simulink model "IntegrationTestSim"  (R2018b)
settings: Solver=ode45  StartTime=0.0  StopTime=600  RelTol=1e-3  EnableMultiTasking=on
values from neighbouring files (symbols this model uses):
  enableHorzMan = 1    [IntegrationTestClass.m]
  enableVertMan = 0    [IntegrationTestClass.m]
  ignorePrevAlert = 1    [IntegrationTestClass.m]
  sim_sampleTime = 0.1    [IntegrationTestClass.m]
  uasSensorSelected = 1    [IntegrationTestClass.m]
  uasSurveillance_sampleTime = 0.1    [IntegrationTestClass.m]
undefined symbols (not defined in the file or in its folder): ac1dyn_alt0_ft, ac1dyn_lat0_rad, ac1dyn_lon0_rad, daa_turnRate_dps, daa_vertRate_fpm, dh_flag, dh_ftps, dpsi_flag, dpsi_radps, uasPilot_altitudeK, uasPilot_altitudeOffset, uasPilot_altitudeTheta, uasPilot_coordDelayK, uasPilot_coordDelayMin, uasPilot_coordDelayTheta, uasPilot_desiredTurnRate_dps, uasPilot_desiredVertRate_ftpm, uasPilot_deterministicMode, uasPilot_dt_s, uasPilot_executionDelayMin, uasPilot_executionDelayMu, uasPilot_initialDelayMin, uasPilot_initialDelayMu, uasPilot_maxRelativeHdg, uasPilot_meanUpdateTimes, uasPilot_mentalFilter_climbThresh_fps, uasPilot_mentalFilter_numSamp, uasPilot_mentalFilter_turnThresh_rad, uasPilot_minUpdateTimes, uasPilot_operatorEnabled, uasPilot_probDescend, uasPilot_probFollowMinDev, uasPilot_probLeftTurn, uasPilot_probTurn, uasPilot_reducedClimbAlt_ft, uasPilot_reducedTurnAngle_deg, uasPilot_seedChoose, uasPilot_seedCoordDelay, uasPilot_seedExecutionDelay, uasPilot_seedInitialDelay, uasPilot_seedTurn, uasPilot_seedUpdate, uasPilot_seedVertical, uasPilot_triggerLevel, uasPilot_turnK, uasPilot_turnOffset, uasPilot_turnTheta
libraries: simulink x4, BasicAircraftDynamicsBlock x3, NominalTrajectory x2, FlattenAircraftEstimateBus x2, PerfectSurveillanceBlock x2, sph2cart x2, DaidalusV201Block x1, HysteresisFilterBlock x1, MofNFilterBlock x1, CommonMetricsBlock x1, SLoWCBlock x1, WellClearMetricsBlock x1
(part 2 of 3)

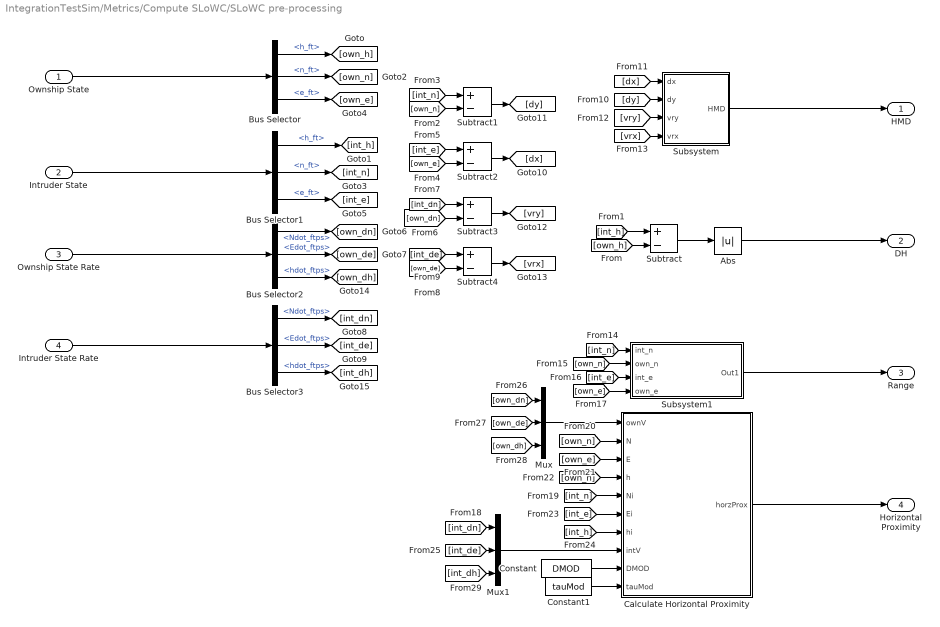
== system IntegrationTestSim/Metrics/Compute SLoWC/SLoWC pre-processing ==
  Ownship State : Inport
  Intruder State : Inport  Port=2
  Ownship State Rate : Inport  Port=3
  Intruder State Rate : Inport  Port=4
  Abs : Abs
  Bus Selector : BusSelector  OutputSignals=h_ft,n_ft,e_ft
  Bus Selector1 : BusSelector  OutputSignals=h_ft,n_ft,e_ft
  Bus Selector2 : BusSelector  OutputSignals=Ndot_ftps,Edot_ftps,hdot_ftps
  Bus Selector3 : BusSelector  OutputSignals=Ndot_ftps,Edot_ftps,hdot_ftps
  Calculate Horizontal Proximity : MATLAB Function  TreatAsAtomicUnit=on
  Constant : Constant  Value=DMOD
  Constant1 : Constant  Value=tauMod
  Mux : Mux  Inputs=3
  Mux1 : Mux  Inputs=3
  Subsystem : Subsystem
  Subsystem1 : Subsystem
  Subtract{,1..4} (5 alike) : Sum  Inputs=+-
  HMD : Outport
  DH : Outport  Port=2
  Range : Outport  Port=3
  Horizontal Proximity : Outport  Port=4
  wires:
  Subtract/1 -> Abs/1
  [own_dh] -> Mux/3
  Bus Selector/1 -> [own_h]  "<h_ft>"
  [own_dn] -> Subtract3/2
  Bus Selector1/3 -> [int_e]  "<e_ft>"
  [int_n] -> Calculate Horizontal Proximity/5(Ni)
  Bus Selector3/3 -> [int_dh]  "<hdot_ftps>"
  [int_h] -> Calculate Horizontal Proximity/7(hi)
  [int_e] -> Subtract2/1
  [own_h] -> Subtract/2
  Intruder State/1 -> Bus Selector1/1
  [own_n] -> Subtract1/2
  Constant/1 -> Calculate Horizontal Proximity/9(DMOD)
  [own_e] -> Subtract2/2
  [int_dh] -> Mux1/3
  Subtract4/1 -> [vrx]
  [int_h] -> Subtract/1
  Bus Selector1/1 -> [int_h]  "<h_ft>"
  [vry] -> Subsystem/3(vry)
  [own_n] -> Calculate Horizontal Proximity/2(N)
  Bus Selector3/1 -> [int_dn]  "<Ndot_ftps>"
  Subtract2/1 -> [dx]
  Bus Selector1/2 -> [int_n]  "<n_ft>"
  Bus Selector/2 -> [own_n]  "<n_ft>"
  Subtract3/1 -> [vry]
  [int_e] -> Subsystem1/3(int_e)
  [own_de] -> Mux/2
  Mux1/1 -> Calculate Horizontal Proximity/8(intV)
  Subtract1/1 -> [dy]
  [own_h] -> Calculate Horizontal Proximity/4(h)
  [dy] -> Subsystem/2(dy)
  [own_n] -> Subsystem1/2(own_n)
  [int_dn] -> Mux1/1
  Subsystem/1(HMD) -> HMD/1
  Bus Selector2/2 -> [own_de]  "<Edot_ftps>"
  [int_n] -> Subtract1/1
  Bus Selector2/3 -> [own_dh]  "<hdot_ftps>"
  [int_de] -> Subtract4/1
  Constant1/1 -> Calculate Horizontal Proximity/10(tauMod)
  Bus Selector/3 -> [own_e]  "<e_ft>"
  Subsystem1/1(Out1) -> Range/1
  [int_n] -> Subsystem1/1("int_n ")
  [int_e] -> Calculate Horizontal Proximity/6(Ei)
  [own_de] -> Subtract4/2
  Bus Selector3/2 -> [int_de]  "<Edot_ftps>"
  Mux/1 -> Calculate Horizontal Proximity/1(ownV)
  [dx] -> Subsystem/1("dx ")
  [int_dn] -> Subtract3/1
  Intruder State Rate/1 -> Bus Selector3/1
  [vrx] -> Subsystem/4(vrx)
  [own_dn] -> Mux/1
  Bus Selector2/1 -> [own_dn]  "<Ndot_ftps>"
  Abs/1 -> DH/1
  [own_e] -> Calculate Horizontal Proximity/3(E)
  Calculate Horizontal Proximity/1(horzProx) -> Horizontal Proximity/1
  Ownship State/1 -> Bus Selector/1
  [int_de] -> Mux1/2
  [own_e] -> Subsystem1/4(own_e)
  Ownship State Rate/1 -> Bus Selector2/1

== system IntegrationTestSim/Pilot/Format Maneuver As AircraftCommand/Get Previous Command ==
  Cmd In : Inport
  Nominal Cmd : Inport  Port=2
  Maneuver Flag : Inport  Port=3
  Data Type Conversion : DataTypeConversion  OutDataTypeStr=double
  Memory : Memory  InheritSampleTime=on
  Switch : Switch  Criteria=u2 > Threshold
  Cmd Out : Outport
  wires:
  Maneuver Flag/1 -> Memory/1
  Memory/1 -> Data Type Conversion/1
  Nominal Cmd/1 -> Switch/3
  Switch/1 -> Cmd Out/1
  Cmd In/1 -> Switch/1
  Data Type Conversion/1 -> Switch/2

== system IntegrationTestSim/Pilot/Format Maneuver As AircraftCommand/Horizontal Maneuver ==
  Command In : Inport
  Maneuver : Inport  Port=2
  Own State : Inport  Port=3
  Maneuver Flag : Inport  Port=4  OutDataTypeStr=boolean
  Bus Selector : BusSelector  OutputSignals=type
  Compare To Constant : simulink/Logic and Bit Operations/Compare To Constant  relop===  const=1  OutDataTypeStr=boolean
  Data Type Conversion1 : DataTypeConversion  OutDataTypeStr=double
  Logical Operator : Logic  AllPortsSameDT=off  OutDataTypeStr=boolean
  Set Desired Turn Rate : Subsystem
  Switch : Switch  Criteria=u2 > Threshold
  Cmd Out : Outport
  wires:
  Bus Selector/1 -> Compare To Constant/1  "<type>"
  Maneuver/1 -> Set Desired Turn Rate/2(Maneuver Magnitude), Bus Selector/1
  Own State/1 -> Set Desired Turn Rate/3(Own State)
  Maneuver Flag/1 -> Data Type Conversion1/1
  Logical Operator/1 -> Switch/2
  Command In/1 -> Switch/3, Set Desired Turn Rate/1(Cmd In)
  Data Type Conversion1/1 -> Logical Operator/1
  Compare To Constant/1 -> Logical Operator/2
  Set Desired Turn Rate/1(Cmd Out) -> Switch/1
  Switch/1 -> Cmd Out/1

== system IntegrationTestSim/Pilot/Format Maneuver As AircraftCommand/Vertical Maneuver ==
  Command In : Inport
  Maneuver : Inport  Port=2
  Own State : Inport  Port=3
  Maneuver Flag : Inport  Port=4  OutDataTypeStr=boolean
  UAS Nominal Traj : Inport  Port=5
  Bus Selector1 : BusSelector  OutputSignals=dh_ftps,h_ft
  Bus Selector : BusSelector  OutputSignals=type
  Compare To Constant : simulink/Logic and Bit Operations/Compare To Constant  relop===  const=2  OutDataTypeStr=boolean
  Data Type Conversion1 : DataTypeConversion  OutDataTypeStr=double
  Logical Operator : Logic  AllPortsSameDT=off  OutDataTypeStr=boolean
  Scope : Scope
  Scope1 : Scope
  Set Desired Vertical Rate : Subsystem
  Switch : Switch  Criteria=u2 > Threshold
  Cmd Out : Outport
  wires:
  Bus Selector/1 -> Compare To Constant/1  "<type>"
  Maneuver Flag/1 -> Data Type Conversion1/1
  Switch/1 -> Cmd Out/1
  Data Type Conversion1/1 -> Logical Operator/1
  Compare To Constant/1 -> Logical Operator/2
  Command In/1 -> Set Desired Vertical Rate/1(Cmd In), Switch/3
  Set Desired Vertical Rate/1(Cmd Out) -> Switch/1
  UAS Nominal Traj/1 -> Bus Selector1/1
  Bus Selector1/2 -> Scope/1  "<h_ft>"
  Own State/1 -> Set Desired Vertical Rate/2(Own State)
  Maneuver/1 -> Set Desired Vertical Rate/3(Maneuver), Bus Selector/1
  Bus Selector1/1 -> Set Desired Vertical Rate/4(dh_ftps)  "<dh_ftps>"
  Logical Operator/1 -> Scope1/1, Switch/2

== system IntegrationTestSim/Pilot/Trigger/Filter Alerts ==
  Alert Level In : Inport
  Constant6 : Constant  Value=trigger_level
  Relational Operator : RelationalOperator  OutDataTypeStr=boolean  RndMeth=Nearest
  Trigger : Outport
  wires:
  Relational Operator/1 -> Trigger/1
  Constant6/1 -> Relational Operator/2
  Alert Level In/1 -> Relational Operator/1

== system IntegrationTestSim/Surveillance Source/Subsystem/EOIR Parameteric Model ==
  Intruder Aircraft State : Inport
  Intruder Aircraft State Rate : Inport  Port=2
  Ownship Aircraft State : Inport  Port=3
  Ownship Aircraft State Rate : Inport  Port=4
  EOIR Parametric Model : EOIRParametricModelBlock/EOIR Parametric Model  dt_s=ac1IntEOIR_dt_s  lat0_rad=ac1dyn_lat0_rad  lon0_rad=ac1dyn_lon0_rad  alt0_ft=ac1dyn_alt0_ft  sns_max_range_ft=ac1IntEOIR_sns_max_range_ft  sns_for_azimuth_deg=ac1IntEOIR_sns_for_azimuth_deg  sns_for_elevation_deg=ac1IntEOIR_sns_for_elevation_deg  rng_random_stddev_ft=ac1IntEOIR_rng_random_stddev_ft  rng_bias_ft=ac1IntEOIR_rng_bias_ft  rng_tau_s=ac1IntEOIR_rng_tau_s  seed1=ac1IntEOIR_seed1  rng_std_dev_gain=ac1IntEOIR_rng_std_dev_gain  rng_bias_switch=ac1IntEOIR_rng_bias_switch  coloredNoiseFlag=0  az_random_stddev_rad=ac1IntEOIR_az_random_stddev_rad  az_bias_rad=ac1IntEOIR_az_bias_rad  az_tau_s=ac1IntEOIR_az_tau_s  seed2=ac1IntEOIR_seed2  el_random_stddev_rad=ac1IntEOIR_el_random_stddev_rad  el_bias_rad=ac1IntEOIR_el_bias_rad  el_tau_s=ac1IntEOIR_el_tau_s  seed3=ac1IntEOIR_seed3  rngdot_random_stddev_ftps=ac1IntEOIR_rngdot_random_stddev_ftps  rngdot_bias_ftps=ac1IntEOIR_rngdot_bias_ftps  rngdot_tau_s=ac1IntEOIR_rngdot_tau_s  seed4=ac1IntEOIR_seed4  rngdot_std_dev_gain=ac1IntEOIR_rngdot_std_dev_gain  rngdot_delay_s=ac1IntEOIR_rngdot_delay_s  azdot_random_stddev_radps=ac1IntEOIR_azdot_random_stddev_radps  azdot_bias_radps=ac1IntEOIR_azdot_bias_radps  azdot_tau_s=ac1IntEOIR_azdot_tau_s  seed5=ac1IntEOIR_seed5  eldot_random_stddev_radps=ac1IntEOIR_eldot_random_stddev_radps  eldot_bias_radps=ac1IntEOIR_eldot_bias_radps  eldot_tau_s=ac1IntEOIR_eldot_tau_s  seed6=ac1IntEOIR_seed6  covRAE=ac1IntEOIR_reported_errorCovRAE
  Terminator : Terminator
  Intruder AircraftEstimate : Outport
  wires:
  Ownship Aircraft State Rate/1 -> EOIR Parametric Model/4
  Intruder Aircraft State/1 -> EOIR Parametric Model/1
  EOIR Parametric Model/1 -> Intruder AircraftEstimate/1
  Intruder Aircraft State Rate/1 -> EOIR Parametric Model/2
  Ownship Aircraft State/1 -> EOIR Parametric Model/3
  EOIR Parametric Model/2 -> Terminator/1

== system IntegrationTestSim/Surveillance Source/Subsystem/Perfect Surveillance ==
  Intruder Aircraft State : Inport
  Intruder Aircraft State Rate : Inport  Port=2
  Intruder Sensor - Perfect Surveillance : PerfectSurveillanceBlock/Perfect Surveillance  Description=|  dt=ac1IntPerfSurv_surveillanceSampletime_s
      | Documentation for Perfect Observation Block                                                                                                                                                                                                                                                                                                                                                                                                          
      |                                                                                                                                                                                                                                                                                                                                                                                                                                                      
      | Description:  The perfect observation block, also known as a perfect                                                                                                                                                                                                                                                                                                                                                                                 
      | surveillance block, receives an Aircraft State, nominally from a Basic                                                                                                                                                                                                                                                                                                                                                                               
      | Aircraft Dynamics block, and outputs an Aircraft Estimate.  The Aircraft                                                                                                                                                                                                                                                                                                                                                                             
      | State that is received as input consists of Latitude, Longitude, and                                                                                                                                                                                                                                                                                                                                                                                 
      | Altitude state information as well as the aircraft position in local                                                                                                                                                                                                                                                                                                                                                                                 
      | coordinates in units of feet for north, east, and height.  The Aircraft                                                                                                                                                                                                                                                                                                                                                                              
      | Estimate outputs consist of estimates for the aircraft Latitude, Longitude, and Altitude, the east, north up position, and sensor covariance.  For perfect surveillance, the covariance estimates are all set to zero as default.  In addition, "time of validity" and a Boolean flag for the sensor report, "is Valid", are outputted as part of the Aircraft Estimate.                                                                             
      |                                                                                                                                                                                                                                                                                                                                                                                                                                                      
      | The initial perfect surveillance block developed receives the aircraft state information from the "AC2 - Basic Aircraft Dynamics" block within the "nominalEncounter" study.  Since the expected output from the AC1 and AC2 aircraft states have slightly different output parameters than what is provided from the perfect surveillance block (i.e., covariance estimates, isValid, and time of validity), the perfect surveillance block         
      | AircraftEstimate output has been left disconnected.                                                                                                                                                                                                                                                                                                                                                                                                  
      |                                                                                                                                                                                                                                                                                                                                                                                                                                                      
      | The initial unit test performed for this perfect observation block was to                                                                                                                                                                                                                                                                                                                                                                            
      | run the nominalEncounter study and to ensure that the simulation completes and no exceptions are encountered.  This unit test was successful (other than receiving a warning that the output of the perfect surveillance block is not connected, which was expected).  A more comprehensive future unit test would be to evaluate the position inputs and compare them with the position outputs to ensure that they are consistent with one another.
  Terminator : Terminator
  Intruder AircraftEstimate : Outport
  wires:
  Intruder Aircraft State/1 -> Intruder Sensor - Perfect Surveillance/1
  Intruder Sensor - Perfect Surveillance/2 -> Terminator/1
  Intruder Aircraft State Rate/1 -> Intruder Sensor - Perfect Surveillance/2
  Intruder Sensor - Perfect Surveillance/1 -> Intruder AircraftEstimate/1

== system IntegrationTestSim/Surveillance Source/Subsystem/SC-228 ADSB Model ==
  Intruder Aircraft State : Inport
  Intruder Aircraft State Rate : Inport  Port=2
  Owship Aircraft State : Inport  Port=3
  SC-228 Sensor Model: ADS-B : ADSB_Block/SC-228 Sensor Model: ADS-B  var_prefix=int_  dt_s=uas_adsb_dt_s  lat0_rad=ac1dyn_lat0_rad  lon0_rad=ac1dyn_lon0_rad  alt0_ft=ac1dyn_alt0_ft  avionicsSeed=uas_adsb_avionicsSeed  N_random_stddev_ft=uas_adsb_N_random_stddev_ft  N_bias_ft=uas_adsb_N_bias_ft  N_tau_s=uas_adsb_N_tau_s  seed1=uas_adsb_seed1  E_random_stddev_ft=uas_adsb_E_random_stddev_ft  E_bias_ft=uas_adsb_E_bias_ft  E_tau_s=uas_adsb_E_tau_s  seed2=uas_adsb_seed2  Ndot_random_stddev_ftps=uas_adsb_Ndot_random_stddev_ftps  Ndot_bias_ftps=uas_adsb_Ndot_bias_ftps  Ndot_tau_s=uas_adsb_Ndot_tau_s  seed5=uas_adsb_seed5  Edot_random_stddev_ftps=uas_adsb_Edot_random_stddev_ftps  Edot_bias_ftps=uas_adsb_Edot_bias_ftps  Edot_tau_s=uas_adsb_Edot_tau_s  seed6=uas_adsb_seed6  covNED=uas_adsb_reported_errorCovNED  perfect=uas_adsb_usePerfectAlt  seed3=uas_adsb_seed3  seed4=uas_adsb_seed4  altQuant_ft=uas_adsb_altQuant_ft  seed7=uas_adsb_seed7  sns_max_range_ft=uas_adsb_sns_max_range_ft  probOneHit_3sec=uas_adsb_probOneHit_3sec  probOneHit_7sec=uas_adsb_probOneHit_7sec  randProbSeed=uas_adsb_randProbSeed  rangeThreshold_ft=uas_adsb_rangeThreshold_ft
  Terminator : Terminator
  Intruder AircraftEstimate : Outport
  wires:
  Owship Aircraft State/1 -> SC-228 Sensor Model: ADS-B/3
  SC-228 Sensor Model: ADS-B/2 -> Terminator/1
  Intruder Aircraft State Rate/1 -> SC-228 Sensor Model: ADS-B/2
  Intruder Aircraft State/1 -> SC-228 Sensor Model: ADS-B/1
  SC-228 Sensor Model: ADS-B/1 -> Intruder AircraftEstimate/1

== system IntegrationTestSim/Surveillance Source/Subsystem/SC-228 ADSB Model (Tracked) ==
  Intruder Aircraft State : Inport
  Intruder Aircraft State Rate : Inport  Port=2
  Ownship Aircraft State : Inport  Port=3
  SC-228 Sensor Model: ADS-B (Tracked) : Tracked_ADSB_Block/SC-228 Sensor Model: ADS-B (Tracked)  var_prefix=int_  dt_s=uas_adsb_trckd_dt_s  lat0_rad=ac1dyn_lat0_rad  lon0_rad=ac1dyn_lon0_rad  alt0_ft=ac1dyn_alt0_ft  avionicsSeed=uas_adsb_trckd_avionicsSeed  N_random_stddev_ft=uas_adsb_trckd_N_stddev_ft  N_bias_ft=uas_adsb_trckd_N_bias_ft  N_tau_s=uas_adsb_trckd_N_tau_s  seed1=uas_adsb_trckd_seed1  E_random_stddev_ft=uas_adsb_trckd_E_stddev_ft  E_bias_ft=uas_adsb_trckd_E_bias_ft  E_tau_s=uas_adsb_trckd_E_tau_s  seed2=uas_adsb_trckd_seed2  Ndot_random_stddev_ftps=uas_adsb_trckd_Ndot_stddev_ftps  Ndot_bias_ftps=uas_adsb_trckd_Ndot_bias_ftps  Ndot_tau_s=uas_adsb_trckd_Ndot_tau_s  seed5=uas_adsb_trckd_seed5  Edot_random_stddev_ftps=uas_adsb_trckd_Edot_stddev_ftps  Edot_bias_ftps=uas_adsb_trckd_Edot_bias_ftps  Edot_tau_s=uas_adsb_trckd_Edot_tau_s  seed6=uas_adsb_trckd_seed6  covNED=uas_adsb_trckd_reported_errorCovNED  seed3=uas_adsb_trckd_seed3  seed4=uas_adsb_trckd_seed4  altQuant_ft=uas_adsb_trckd_altQuant_ft  seed7=uas_adsb_trckd_seed7  sns_max_range_ft=uas_adsb_trckd_sns_max_range_ft  probOneHit_3sec=uas_adsb_trckd_probOneHit_3sec  probOneHit_7sec=uas_adsb_trckd_probOneHit_7sec  randProbSeed=uas_adsb_trckd_randProbSeed  rangeThreshold_ft=uas_adsb_trckd_rangeThreshold_ft
  Intruder AircraftEstimate : Outport
  wires:
  SC-228 Sensor Model: ADS-B (Tracked)/1 -> Intruder AircraftEstimate/1
  Ownship Aircraft State/1 -> SC-228 Sensor Model: ADS-B (Tracked)/3
  Intruder Aircraft State Rate/1 -> SC-228 Sensor Model: ADS-B (Tracked)/2
  Intruder Aircraft State/1 -> SC-228 Sensor Model: ADS-B (Tracked)/1

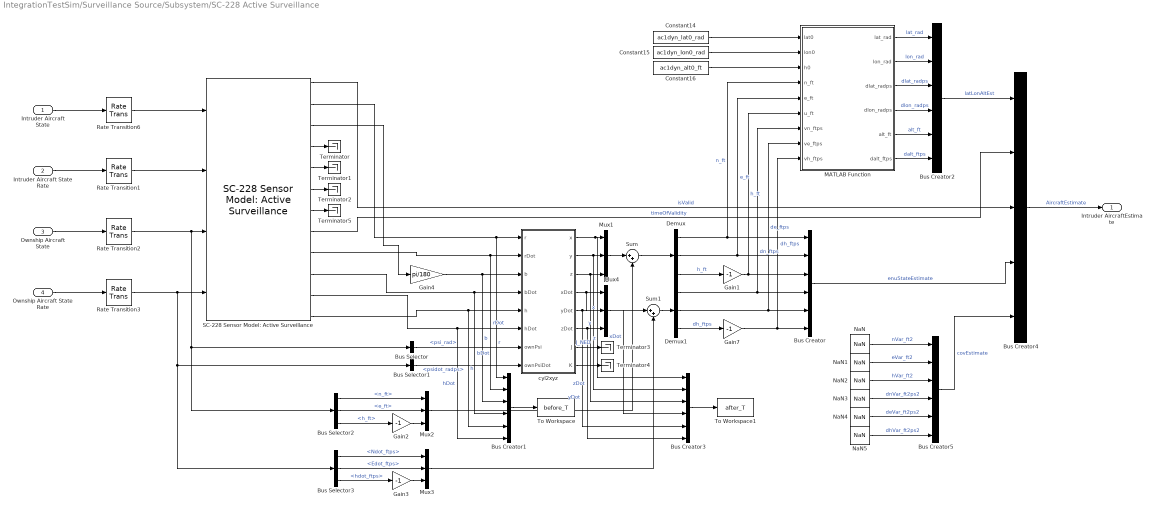
== system IntegrationTestSim/Surveillance Source/Subsystem/SC-228 Active Surveillance ==
  Intruder Aircraft State : Inport
  Intruder Aircraft State Rate : Inport  Port=2
  Ownship Aircraft State : Inport  Port=3
  Ownship Aircraft State Rate : Inport  Port=4
  Bus Creator : BusCreator  Inputs=6  OutDataTypeStr=Bus: StateEstimate
  Bus Creator1 : BusCreator  Inputs=6
  Bus Creator2 : BusCreator  Inputs=6  OutDataTypeStr=Bus: LatLonAltMeasurement
  Bus Creator3 : BusCreator  Inputs=6
  Bus Creator4 : BusCreator  Inputs='latLonAltEst','timeOfValidity','isValid','enuStateEstimate','covEstimate'  OutDataTypeStr=Bus: AircraftEstimate  NonVirtualBus=on
  Bus Creator5 : BusCreator  Inputs=6  OutDataTypeStr=Bus: CovarianceEstimate
  Bus Selector : BusSelector  OutputSignals=psi_rad
  Bus Selector1 : BusSelector  OutputSignals=psidot_radps
  Bus Selector2 : BusSelector  OutputSignals=n_ft,e_ft,h_ft
  Bus Selector3 : BusSelector  OutputSignals=Ndot_ftps,Edot_ftps,hdot_ftps
  Constant14 : Constant  Value=ac1dyn_lat0_rad  OutDataTypeStr=double  SampleTime=sim_sampleTime
  Constant15 : Constant  Value=ac1dyn_lon0_rad  OutDataTypeStr=double  SampleTime=sim_sampleTime
  Constant16 : Constant  Value=ac1dyn_alt0_ft  OutDataTypeStr=double  SampleTime=sim_sampleTime
  Demux : Demux  Outputs=3
  Demux1 : Demux  Outputs=3
  Gain{1..3,7} (4 alike) : Gain  Gain=-1
  Gain4 : Gain  Gain=pi/180
  MATLAB Function : MATLAB Function  TreatAsAtomicUnit=on
  Mux{1..4} (4 alike) : Mux  Inputs=3
  NaN{,1..5} (6 alike) : Constant  Value=NaN  OutDataTypeStr=Inherit: Inherit via back propagation
  Rate Transition{1..3,6} (4 alike) : RateTransition  OutPortSampleTime=uasLogic_sampleTime
  SC-228 Sensor Model: Active Surveillance : ActiveSurveillance_Block/SC-228 Sensor Model: Active Surveillance  dt_s=uas_tcas_dt_s  lat0_rad=ac1dyn_lat0_rad  lon0_rad=ac1dyn_lon0_rad  alt0_ft=ac1dyn_alt0_ft  sns_max_range_ft=uas_tcas_sns_max_range_ft  rng_random_stddev_ft=uas_tcas_rng_random_stddev_ft  rng_bias_ft=uas_tcas_rng_bias_ft  rng_tau_s=uas_tcas_rng_tau_s  seed1=uas_tcas_seed1  bearing_Max_deg=uas_tcas_bearing_Max_deg  bearing_Sigma_deg=uas_tcas_bearing_Sigma_deg  bearing_Breakpoints_deg=uas_tcas_bearing_Breakpoints_deg  seed2=uas_tcas_seed2  seed3=uas_tcas_seed3  seed4=uas_tcas_seed4  altQuant_ft=uas_tcas_altQuant_ft  covRBA=uas_tcas_reported_errorCovRBA  sns_max_front_range_ft=uas_tcas_sns_max_front_range_ft  sns_max_side_range_ft=uas_tcas_sns_max_side_range_ft  sns_max_rear_range_ft=uas_tcas_sns_max_rear_range_ft  probDetect=uas_tcas_probDetect  FOR_elev_max_deg=uas_tcas_FOR_elev_max_deg  FOR_elev_min_deg=uas_tcas_FOR_elev_min_deg  randProbSeed=uas_tcas_randProbSeed  tauThreshold_sec=uas_tcas_tauThreshold_sec  updateRate_sec=uas_tcas_updateRate_sec
  Sum : Sum  Inputs=|++
  Sum1 : Sum  Inputs=|++
  Terminator{,1..5} (6 alike) : Terminator
  To Workspace : ToWorkspace  VariableName=before_T  SaveFormat=Timeseries  SampleTime=-1
  To Workspace1 : ToWorkspace  VariableName=after_T  SaveFormat=Timeseries  SampleTime=-1
  cyl2xyz : MATLAB Function  TreatAsAtomicUnit=on
  Intruder AircraftEstimate : Outport
  wires:
  SC-228 Sensor Model: Active Surveillance/6 -> Terminator2/1
  SC-228 Sensor Model: Active Surveillance/7 -> Terminator5/1
  SC-228 Sensor Model: Active Surveillance/4 -> Terminator/1
  SC-228 Sensor Model: Active Surveillance/5 -> Terminator1/1
  Intruder Aircraft State/1 -> Rate Transition6/1
  Intruder Aircraft State Rate/1 -> Rate Transition1/1
  Gain1/1 -> MATLAB Function/6(u_ft), Bus Creator/3  "h_ft"
  Gain7/1 -> MATLAB Function/9(vh_ftps), Bus Creator/6  "dh_ftps"
  cyl2xyz/3(z) -> Bus Creator3/3, Mux1/3  "z"
  Sum1/1 -> Demux1/1
  cyl2xyz/5(yDot) -> Mux4/2, Bus Creator3/5  "yDot"
  Bus Selector/1 -> cyl2xyz/7(ownPsi)  "<psi_rad>"
  cyl2xyz/4(xDot) -> Bus Creator3/4, Mux4/1  "xDot"
  cyl2xyz/6(zDot) -> Bus Creator3/6, Mux4/3  "zDot"
  Demux/2 -> MATLAB Function/5(e_ft), Bus Creator/2  "e_ft"
  Bus Selector2/3 -> Gain2/1  "<h_ft>"
  cyl2xyz/7(J) -> Terminator3/1  "J_NED"
  Mux1/1 -> Sum/1
  Sum/1 -> Demux/1
  Demux/1 -> MATLAB Function/4(n_ft), Bus Creator/1  "n_ft"
  Mux2/1 -> Sum/2
  Ownship Aircraft State Rate/1 -> Rate Transition3/1
  Bus Selector1/1 -> cyl2xyz/8(ownPsiDot)  "<psidot_radps>"
  cyl2xyz/2(y) -> Bus Creator3/2, Mux1/2  "y"
  Demux1/3 -> Gain7/1  "dh_ftps"
  Demux1/2 -> MATLAB Function/8(ve_ftps), Bus Creator/5  "de_ftps"
  Gain2/1 -> Mux2/3
  Gain3/1 -> Mux3/3
  SC-228 Sensor Model: Active Surveillance/3 -> Gain4/1
  SC-228 Sensor Model: Active Surveillance/10 -> Bus Creator1/4, cyl2xyz/4(bDot)  "bDot"
  Bus Selector2/2 -> Mux2/2  "<e_ft>"
  Demux/3 -> Gain1/1  "h_ft"
  Gain4/1 -> Bus Creator1/3, cyl2xyz/3(b)  "b"
  Mux3/1 -> Sum1/2
  Demux1/1 -> MATLAB Function/7(vn_ftps), Bus Creator/4  "dn_ftps"
  SC-228 Sensor Model: Active Surveillance/11 -> Bus Creator1/6, cyl2xyz/6(hDot)  "hDot"
  Bus Creator/1 -> Bus Creator4/4  "enuStateEstimate"
  Bus Selector3/1 -> Mux3/1  "<Ndot_ftps>"
  Bus Selector2/1 -> Mux2/1  "<n_ft>"
  SC-228 Sensor Model: Active Surveillance/9 -> Bus Creator1/2, cyl2xyz/2(rDot)  "rDot"
  Bus Selector3/2 -> Mux3/2  "<Edot_ftps>"
  cyl2xyz/1(x) -> Bus Creator3/1, Mux1/1  "x"
  Bus Selector3/3 -> Gain3/1  "<hdot_ftps>"
  SC-228 Sensor Model: Active Surveillance/2 -> Bus Creator1/1, cyl2xyz/1(r)  "r"
  SC-228 Sensor Model: Active Surveillance/12 -> Bus Creator1/5, cyl2xyz/5(h)  "h"
  Mux4/1 -> Sum1/1
  Ownship Aircraft State/1 -> Rate Transition2/1
  SC-228 Sensor Model: Active Surveillance/8 -> Bus Creator4/2  "timeOfValidity"
  NaN1/1 -> Bus Creator5/2  "eVar_ft2"
  Constant16/1 -> MATLAB Function/3(h0)
  MATLAB Function/5(alt_ft) -> Bus Creator2/5  "alt_ft"
  Bus Creator2/1 -> Bus Creator4/1  "latLonAltEst"
  Constant14/1 -> MATLAB Function/1(lat0)
  Bus Creator5/1 -> Bus Creator4/5  "covEstimate"
  MATLAB Function/6(dalt_ftps) -> Bus Creator2/6  "dalt_ftps"
  MATLAB Function/1(lat_rad) -> Bus Creator2/1  "lat_rad"
  Constant15/1 -> MATLAB Function/2(lon0)
  MATLAB Function/3(dlat_radps) -> Bus Creator2/3  "dlat_radps"
  Bus Creator4/1 -> Intruder AircraftEstimate/1  "AircraftEstimate"
  MATLAB Function/4(dlon_radps) -> Bus Creator2/4  "dlon_radps"
  NaN5/1 -> Bus Creator5/6  "dhVar_ft2ps2"
  NaN2/1 -> Bus Creator5/3  "hVar_ft2"
  NaN/1 -> Bus Creator5/1  "nVar_ft2"
  NaN4/1 -> Bus Creator5/5  "deVar_ft2ps2"
  MATLAB Function/2(lon_rad) -> Bus Creator2/2  "lon_rad"
  NaN3/1 -> Bus Creator5/4  "dnVar_ft2ps2"
  SC-228 Sensor Model: Active Surveillance/1 -> Bus Creator4/3  "isValid"
  Rate Transition6/1 -> SC-228 Sensor Model: Active Surveillance/1
  Rate Transition1/1 -> SC-228 Sensor Model: Active Surveillance/2
  Rate Transition2/1 -> SC-228 Sensor Model: Active Surveillance/3, Bus Selector/1, Bus Selector2/1
  Rate Transition3/1 -> SC-228 Sensor Model: Active Surveillance/4, Bus Selector1/1, Bus Selector3/1
  Bus Creator1/1 -> To Workspace/1
  Bus Creator3/1 -> To Workspace1/1
  cyl2xyz/8(K) -> Terminator4/1

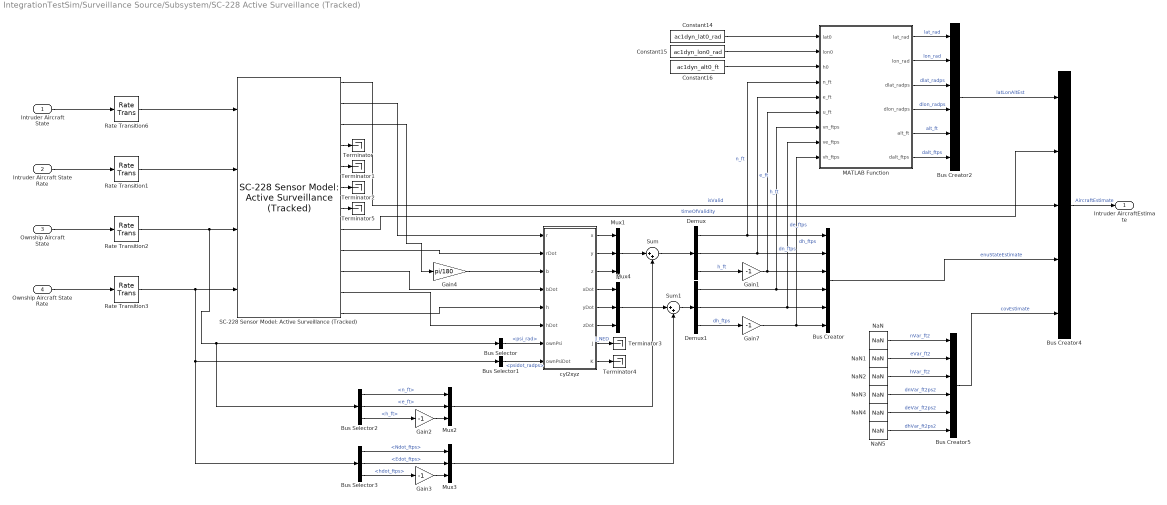
== system IntegrationTestSim/Surveillance Source/Subsystem/SC-228 Active Surveillance (Tracked) ==
  Intruder Aircraft State : Inport
  Intruder Aircraft State Rate : Inport  Port=2
  Ownship Aircraft State : Inport  Port=3
  Ownship Aircraft State Rate : Inport  Port=4
  Bus Creator : BusCreator  Inputs=6  OutDataTypeStr=Bus: StateEstimate
  Bus Creator2 : BusCreator  Inputs=6  OutDataTypeStr=Bus: LatLonAltMeasurement
  Bus Creator4 : BusCreator  Inputs='latLonAltEst','timeOfValidity','isValid','enuStateEstimate','covEstimate'  OutDataTypeStr=Bus: AircraftEstimate  NonVirtualBus=on
  Bus Creator5 : BusCreator  Inputs=6  OutDataTypeStr=Bus: CovarianceEstimate
  Bus Selector : BusSelector  OutputSignals=psi_rad
  Bus Selector1 : BusSelector  OutputSignals=psidot_radps
  Bus Selector2 : BusSelector  OutputSignals=n_ft,e_ft,h_ft
  Bus Selector3 : BusSelector  OutputSignals=Ndot_ftps,Edot_ftps,hdot_ftps
  Constant14 : Constant  Value=ac1dyn_lat0_rad  OutDataTypeStr=double  SampleTime=sim_sampleTime
  Constant15 : Constant  Value=ac1dyn_lon0_rad  OutDataTypeStr=double  SampleTime=sim_sampleTime
  Constant16 : Constant  Value=ac1dyn_alt0_ft  OutDataTypeStr=double  SampleTime=sim_sampleTime
  Demux : Demux  Outputs=3
  Demux1 : Demux  Outputs=3
  Gain{1..3,7} (4 alike) : Gain  Gain=-1
  Gain4 : Gain  Gain=pi/180
  MATLAB Function : MATLAB Function  TreatAsAtomicUnit=on
  Mux{1..4} (4 alike) : Mux  Inputs=3
  NaN{,1..5} (6 alike) : Constant  Value=NaN  OutDataTypeStr=Inherit: Inherit via back propagation
  Rate Transition{1..3,6} (4 alike) : RateTransition  OutPortSampleTime=uasLogic_sampleTime
  SC-228 Sensor Model: Active Surveillance (Tracked) : Tracked_ActiveSurveillance_Block/SC-228 Sensor Model: Active Surveillance (Tracked)  dt_s=uas_tcas_dt_s  lat0_rad=ac1dyn_lat0_rad  lon0_rad=ac1dyn_lon0_rad  alt0_ft=ac1dyn_alt0_ft  sns_max_range_ft=uas_tcas_trckd_sns_max_range_ft  rng_random_stddev_ft=uas_tcas_trckd_rng_random_stddev_ft  rng_bias_ft=uas_tcas_trckd_rng_bias_ft  rng_tau_s=0  seed1=uas_tcas_trckd_seed1  bearing_Max_deg=uas_tcas_trckd_bearing_Max_deg  bearing_Sigma_deg=uas_tcas_trckd_bearing_Sigma_deg  bearing_Breakpoints_deg=uas_tcas_trckd_bearing_Breakpoints_deg  seed2=uas_tcas_trckd_seed2  seed3=uas_tcas_trckd_seed3  seed4=uas_tcas_trckd_seed4  altQuant_ft=uas_tcas_trckd_altQuant_ft  covRBA=uas_tcas_trckd_reported_errorCovRBA  sns_max_front_range_ft=uas_tcas_trckd_sns_max_front_range_ft  sns_max_side_range_ft=uas_tcas_trckd_sns_max_side_range_ft  sns_max_rear_range_ft=uas_tcas_trckd_sns_max_rear_range_ft  probDetect=uas_tcas_trckd_probDetect  FOR_elev_max_deg=uas_tcas_trckd_FOR_elev_max_deg  FOR_elev_min_deg=uas_tcas_trckd_FOR_elev_min_deg  randProbSeed=uas_tcas_trckd_randProbSeed  tauThreshold_sec=uas_tcas_trckd_tauThreshold_sec  updateRate_sec=uas_tcas_trckd_updateRate_sec
  Sum : Sum  Inputs=|++
  Sum1 : Sum  Inputs=|++
  Terminator{,1..5} (6 alike) : Terminator
  cyl2xyz : MATLAB Function  TreatAsAtomicUnit=on
  Intruder AircraftEstimate : Outport
  wires:
  Intruder Aircraft State Rate/1 -> Rate Transition1/1
  Intruder Aircraft State/1 -> Rate Transition6/1
  cyl2xyz/2(y) -> Mux1/2
  Demux1/2 -> MATLAB Function/8(ve_ftps), Bus Creator/5  "de_ftps"
  Bus Selector1/1 -> cyl2xyz/8(ownPsiDot)  "<psidot_radps>"
  Mux2/1 -> Sum/2
  Demux/1 -> MATLAB Function/4(n_ft), Bus Creator/1  "n_ft"
  Mux1/1 -> Sum/1
  cyl2xyz/8(K) -> Terminator4/1
  Sum/1 -> Demux/1
  cyl2xyz/7(J) -> Terminator3/1  "J_NED"
  Bus Selector2/3 -> Gain2/1  "<h_ft>"
  Demux/2 -> MATLAB Function/5(e_ft), Bus Creator/2  "e_ft"
  cyl2xyz/6(zDot) -> Mux4/3
  cyl2xyz/4(xDot) -> Mux4/1
  Bus Selector/1 -> cyl2xyz/7(ownPsi)  "<psi_rad>"
  Gain7/1 -> MATLAB Function/9(vh_ftps), Bus Creator/6  "dh_ftps"
  cyl2xyz/3(z) -> Mux1/3
  MATLAB Function/6(dalt_ftps) -> Bus Creator2/6  "dalt_ftps"
  MATLAB Function/4(dlon_radps) -> Bus Creator2/4  "dlon_radps"
  SC-228 Sensor Model: Active Surveillance (Tracked)/4 -> Terminator/1
  MATLAB Function/2(lon_rad) -> Bus Creator2/2  "lon_rad"
  NaN1/1 -> Bus Creator5/2  "eVar_ft2"
  Constant16/1 -> MATLAB Function/3(h0)
  SC-228 Sensor Model: Active Surveillance (Tracked)/2 -> cyl2xyz/1(r)
  MATLAB Function/5(alt_ft) -> Bus Creator2/5  "alt_ft"
  Constant14/1 -> MATLAB Function/1(lat0)
  Bus Creator2/1 -> Bus Creator4/1  "latLonAltEst"
  Demux1/3 -> Gain7/1  "dh_ftps"
  NaN/1 -> Bus Creator5/1  "nVar_ft2"
  Ownship Aircraft State Rate/1 -> Rate Transition3/1
  MATLAB Function/1(lat_rad) -> Bus Creator2/1  "lat_rad"
  NaN2/1 -> Bus Creator5/3  "hVar_ft2"
  Sum1/1 -> Demux1/1
  NaN3/1 -> Bus Creator5/4  "dnVar_ft2ps2"
  SC-228 Sensor Model: Active Surveillance (Tracked)/5 -> Terminator1/1
  SC-228 Sensor Model: Active Surveillance (Tracked)/9 -> cyl2xyz/2(rDot)
  Constant15/1 -> MATLAB Function/2(lon0)
  Bus Creator/1 -> Bus Creator4/4  "enuStateEstimate"
  SC-228 Sensor Model: Active Surveillance (Tracked)/3 -> Gain4/1
  NaN5/1 -> Bus Creator5/6  "dhVar_ft2ps2"
  SC-228 Sensor Model: Active Surveillance (Tracked)/11 -> cyl2xyz/6(hDot)
  SC-228 Sensor Model: Active Surveillance (Tracked)/7 -> Terminator5/1
  Mux4/1 -> Sum1/1
  cyl2xyz/5(yDot) -> Mux4/2
  Bus Selector3/3 -> Gain3/1  "<hdot_ftps>"
  NaN4/1 -> Bus Creator5/5  "deVar_ft2ps2"
  cyl2xyz/1(x) -> Mux1/1
  Bus Selector3/2 -> Mux3/2  "<Edot_ftps>"
  Bus Selector2/1 -> Mux2/1  "<n_ft>"
  Bus Selector3/1 -> Mux3/1  "<Ndot_ftps>"
  SC-228 Sensor Model: Active Surveillance (Tracked)/12 -> cyl2xyz/5(h)
  Demux1/1 -> MATLAB Function/7(vn_ftps), Bus Creator/4  "dn_ftps"
  Ownship Aircraft State/1 -> Rate Transition2/1
  Mux3/1 -> Sum1/2
  Gain1/1 -> MATLAB Function/6(u_ft), Bus Creator/3  "h_ft"
  Bus Selector2/2 -> Mux2/2  "<e_ft>"
  SC-228 Sensor Model: Active Surveillance (Tracked)/10 -> cyl2xyz/4(bDot)
  Gain3/1 -> Mux3/3
  Bus Creator4/1 -> Intruder AircraftEstimate/1  "AircraftEstimate"
  Gain4/1 -> cyl2xyz/3(b)
  MATLAB Function/3(dlat_radps) -> Bus Creator2/3  "dlat_radps"
  Demux/3 -> Gain1/1  "h_ft"
  SC-228 Sensor Model: Active Surveillance (Tracked)/6 -> Terminator2/1
  Bus Creator5/1 -> Bus Creator4/5  "covEstimate"
  Gain2/1 -> Mux2/3
  SC-228 Sensor Model: Active Surveillance (Tracked)/8 -> Bus Creator4/2  "timeOfValidity"
  Rate Transition1/1 -> SC-228 Sensor Model: Active Surveillance (Tracked)/2
  Rate Transition6/1 -> SC-228 Sensor Model: Active Surveillance (Tracked)/1
  Rate Transition3/1 -> SC-228 Sensor Model: Active Surveillance (Tracked)/4, Bus Selector1/1, Bus Selector3/1
  Rate Transition2/1 -> SC-228 Sensor Model: Active Surveillance (Tracked)/3, Bus Selector/1, Bus Selector2/1
  SC-228 Sensor Model: Active Surveillance (Tracked)/1 -> Bus Creator4/3  "isValid"

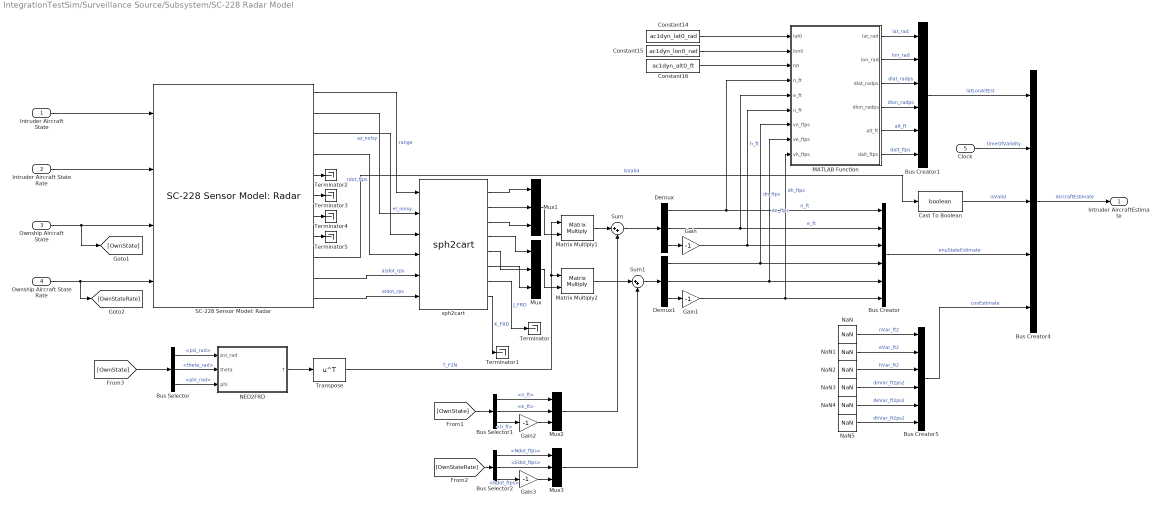
== system IntegrationTestSim/Surveillance Source/Subsystem/SC-228 Radar Model ==
  Intruder Aircraft State : Inport
  Intruder Aircraft State Rate : Inport  Port=2
  Ownship Aircraft State : Inport  Port=3
  Ownship Aircraft State Rate : Inport  Port=4
  Clock : Inport  Port=5
  Bus Creator : BusCreator  Inputs=6  OutDataTypeStr=Bus: StateEstimate
  Bus Creator1 : BusCreator  Inputs=6  OutDataTypeStr=Bus: LatLonAltMeasurement
  Bus Creator4 : BusCreator  Inputs='latLonAltEst','timeOfValidity','isValid','enuStateEstimate','covEstimate'  OutDataTypeStr=Bus: AircraftEstimate  NonVirtualBus=on
  Bus Creator5 : BusCreator  Inputs=6  OutDataTypeStr=Bus: CovarianceEstimate
  Bus Selector : BusSelector  OutputSignals=psi_rad,theta_rad,phi_rad
  Bus Selector1 : BusSelector  OutputSignals=n_ft,e_ft,h_ft
  Bus Selector2 : BusSelector  OutputSignals=Ndot_ftps,Edot_ftps,hdot_ftps
  Cast To Boolean : DataTypeConversion  OutDataTypeStr=boolean
  Constant14 : Constant  Value=ac1dyn_lat0_rad  OutDataTypeStr=double  SampleTime=sim_sampleTime
  Constant15 : Constant  Value=ac1dyn_lon0_rad  OutDataTypeStr=double  SampleTime=sim_sampleTime
  Constant16 : Constant  Value=ac1dyn_alt0_ft  OutDataTypeStr=double  SampleTime=sim_sampleTime
  Demux : Demux  Outputs=3
  Demux1 : Demux  Outputs=3
  Gain{,1..3} (4 alike) : Gain  Gain=-1
  MATLAB Function : MATLAB Function  TreatAsAtomicUnit=on
  Matrix Multiply1 : Product  Multiplication=Matrix(*)
  Matrix Multiply2 : Product  Multiplication=Matrix(*)
  Mux{,1..3} (4 alike) : Mux  Inputs=3
  NED2FRD : MATLAB Function  TreatAsAtomicUnit=on
  NaN{,1..5} (6 alike) : Constant  Value=NaN  OutDataTypeStr=Inherit: Inherit via back propagation
  SC-228 Sensor Model: Radar : Radar_Block/SC-228 Sensor Model: Radar  dt_s=uas_rdr_dt_s  lat0_rad=ac1dyn_lat0_rad  lon0_rad=ac1dyn_lon0_rad  alt0_ft=ac1dyn_alt0_ft  sns_for_azimuth_deg=uas_rdr_sns_for_azimuth_deg  sns_for_elevation_deg=uas_rdr_sns_for_elevation_deg  debugMode=uas_rdr_debugMode  rng_random_stddev_ft=uas_rdr_rng_random_stddev_ft  rng_bias_ft=uas_rdr_rng_bias_ft  rng_tau_s=uas_rdr_rng_tau_s  seed1=uas_rdr_seed1  RCPR_Mode=uas_rdr_RCPR_Mode  RCPR_Range_ft=uas_rdr_RCPR_Range_ft  az_random_stddev_rad=uas_rdr_az_random_stddev_rad  az_bias_rad=uas_rdr_az_bias_rad  az_tau_s=uas_rdr_az_tau_s  seed2=uas_rdr_seed2  el_random_stddev_rad=uas_rdr_el_random_stddev_rad  el_bias_rad=uas_rdr_el_bias_rad  el_tau_s=uas_rdr_el_tau_s  seed3=uas_rdr_seed3  rngdot_random_stddev_ftps=uas_rdr_rngdot_random_stddev_ftps  rngdot_bias_ftps=uas_rdr_rngdot_bias_ftps  rngdot_tau_s=uas_rdr_rngdot_tau_s  seed4=uas_rdr_seed4  covRAE=uas_rdr_reported_errorCovRAE
  Sum : Sum  Inputs=|++
  Sum1 : Sum  Inputs=|++
  Terminator{,1..5} (6 alike) : Terminator
  Transpose : Math  Operator=transpose  SaturateOnIntegerOverflow=on
  sph2cart : sph2cart/sph2cart  SystemSampleTime=-1
      settings: SourceProductName=CASSATTv6: Signals Library
  Intruder AircraftEstimate : Outport
  wires:
  Intruder Aircraft State/1 -> SC-228 Sensor Model: Radar/1
  Intruder Aircraft State Rate/1 -> SC-228 Sensor Model: Radar/2
  Ownship Aircraft State Rate/1 -> [OwnStateRate], SC-228 Sensor Model: Radar/4
  SC-228 Sensor Model: Radar/6 -> Terminator3/1
  SC-228 Sensor Model: Radar/8 -> Terminator5/1
  SC-228 Sensor Model: Radar/7 -> Terminator4/1
  SC-228 Sensor Model: Radar/5 -> Terminator2/1
  [OwnStateRate] -> Bus Selector2/1
  Gain2/1 -> Mux2/3
  Bus Creator5/1 -> Bus Creator4/5  "covEstimate"
  Bus Selector/1 -> NED2FRD/1(psi_rad)  "<psi_rad>"
  Mux3/1 -> Sum1/2
  MATLAB Function/2(lon_rad) -> Bus Creator1/2  "lon_rad"
  NaN3/1 -> Bus Creator5/4  "dnVar_ft2ps2"
  Mux2/1 -> Sum/2
  [OwnState] -> Bus Selector1/1
  Gain3/1 -> Mux3/3
  NaN/1 -> Bus Creator5/1  "nVar_ft2"
  NaN5/1 -> Bus Creator5/6  "dhVar_ft2ps2"
  Bus Selector2/1 -> Mux3/1  "<Ndot_ftps>"
  Bus Creator1/1 -> Bus Creator4/1  "latLonAltEst"
  NED2FRD/1(T) -> Transpose/1
  Sum/1 -> Demux/1
  Bus Selector2/2 -> Mux3/2  "<Edot_ftps>"
  Demux1/3 -> Gain1/1
  NaN2/1 -> Bus Creator5/3  "hVar_ft2"
  Bus Selector/2 -> NED2FRD/2(theta)  "<theta_rad>"
  NaN1/1 -> Bus Creator5/2  "eVar_ft2"
  NaN4/1 -> Bus Creator5/5  "deVar_ft2ps2"
  Matrix Multiply2/1 -> Sum1/1
  MATLAB Function/6(dalt_ftps) -> Bus Creator1/6  "dalt_ftps"
  Bus Selector1/2 -> Mux2/2  "<e_ft>"
  Matrix Multiply1/1 -> Sum/1
  SC-228 Sensor Model: Radar/2 -> sph2cart/2  "az_noisy"
  Demux/3 -> Gain/1
  sph2cart/5 -> Mux/2
  Bus Selector1/1 -> Mux2/1  "<n_ft>"
  Sum1/1 -> Demux1/1
  Bus Selector1/3 -> Gain2/1  "<h_ft>"
  Mux1/1 -> Matrix Multiply1/2
  Gain1/1 -> MATLAB Function/9(vh_ftps), Bus Creator/6  "dh_ftps"
  Bus Creator4/1 -> Intruder AircraftEstimate/1  "AircraftEstimate"
  sph2cart/3 -> Mux1/3
  Constant16/1 -> MATLAB Function/3(h0)
  SC-228 Sensor Model: Radar/10 -> sph2cart/5  "azdot_rps"
  Transpose/1 -> Matrix Multiply2/1, Matrix Multiply1/1  "T_F2N"
  sph2cart/1 -> Mux1/1
  Demux1/2 -> MATLAB Function/8(ve_ftps), Bus Creator/5  "de_ftps"
  sph2cart/6 -> Mux/3
  Bus Selector2/3 -> Gain3/1  "<hdot_ftps>"
  Ownship Aircraft State/1 -> [OwnState], SC-228 Sensor Model: Radar/3
  Demux/1 -> MATLAB Function/4(n_ft), Bus Creator/1  "n_ft"
  MATLAB Function/3(dlat_radps) -> Bus Creator1/3  "dlat_radps"
  Gain/1 -> MATLAB Function/6(u_ft), Bus Creator/3  "h_ft"
  Constant15/1 -> MATLAB Function/2(lon0)
  sph2cart/2 -> Mux1/2
  Mux/1 -> Matrix Multiply2/2
  Demux1/1 -> MATLAB Function/7(vn_ftps), Bus Creator/4  "dn_ftps"
  MATLAB Function/4(dlon_radps) -> Bus Creator1/4  "dlon_radps"
  SC-228 Sensor Model: Radar/4 -> sph2cart/4  "rdot_ftps"
  Bus Creator/1 -> Bus Creator4/4  "enuStateEstimate"
  MATLAB Function/5(alt_ft) -> Bus Creator1/5  "alt_ft"
  SC-228 Sensor Model: Radar/1 -> sph2cart/1  "range"
  Demux/2 -> MATLAB Function/5(e_ft), Bus Creator/2  "e_ft"
  sph2cart/4 -> Mux/1
  Clock/1 -> Bus Creator4/2  "timeOfValidity"
  SC-228 Sensor Model: Radar/3 -> sph2cart/3  "el_noisy"
  Bus Selector/3 -> NED2FRD/3(phi)  "<phi_rad>"
  SC-228 Sensor Model: Radar/11 -> sph2cart/6  "eldot_rps"
  [OwnState] -> Bus Selector/1
  SC-228 Sensor Model: Radar/9 -> Cast To Boolean/1  "isValid"
  sph2cart/7 -> Terminator/1  "J_FRD"
  sph2cart/8 -> Terminator1/1  "K_FRD"
  Constant14/1 -> MATLAB Function/1(lat0)
  MATLAB Function/1(lat_rad) -> Bus Creator1/1  "lat_rad"
  Cast To Boolean/1 -> Bus Creator4/3  "isValid"

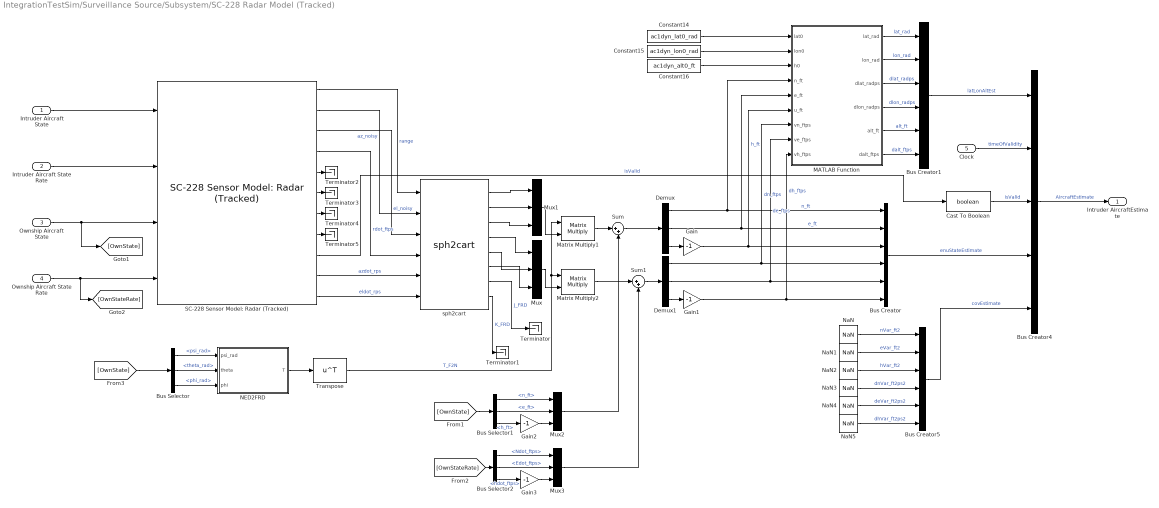
== system IntegrationTestSim/Surveillance Source/Subsystem/SC-228 Radar Model (Tracked) ==
  Intruder Aircraft State : Inport
  Intruder Aircraft State Rate : Inport  Port=2
  Ownship Aircraft State : Inport  Port=3
  Ownship Aircraft State Rate : Inport  Port=4
  Clock : Inport  Port=5
  Bus Creator : BusCreator  Inputs=6  OutDataTypeStr=Bus: StateEstimate
  Bus Creator1 : BusCreator  Inputs=6  OutDataTypeStr=Bus: LatLonAltMeasurement
  Bus Creator4 : BusCreator  Inputs='latLonAltEst','timeOfValidity','isValid','enuStateEstimate','covEstimate'  OutDataTypeStr=Bus: AircraftEstimate  NonVirtualBus=on
  Bus Creator5 : BusCreator  Inputs=6  OutDataTypeStr=Bus: CovarianceEstimate
  Bus Selector : BusSelector  OutputSignals=psi_rad,theta_rad,phi_rad
  Bus Selector1 : BusSelector  OutputSignals=n_ft,e_ft,h_ft
  Bus Selector2 : BusSelector  OutputSignals=Ndot_ftps,Edot_ftps,hdot_ftps
  Cast To Boolean : DataTypeConversion  OutDataTypeStr=boolean
  Constant14 : Constant  Value=ac1dyn_lat0_rad  OutDataTypeStr=double  SampleTime=sim_sampleTime
  Constant15 : Constant  Value=ac1dyn_lon0_rad  OutDataTypeStr=double  SampleTime=sim_sampleTime
  Constant16 : Constant  Value=ac1dyn_alt0_ft  OutDataTypeStr=double  SampleTime=sim_sampleTime
  Demux : Demux  Outputs=3
  Demux1 : Demux  Outputs=3
  Gain{,1..3} (4 alike) : Gain  Gain=-1
  MATLAB Function : MATLAB Function  TreatAsAtomicUnit=on
  Matrix Multiply1 : Product  Multiplication=Matrix(*)
  Matrix Multiply2 : Product  Multiplication=Matrix(*)
  Mux{,1..3} (4 alike) : Mux  Inputs=3
  NED2FRD : MATLAB Function  TreatAsAtomicUnit=on
  NaN{,1..5} (6 alike) : Constant  Value=NaN  OutDataTypeStr=Inherit: Inherit via back propagation
  SC-228 Sensor Model: Radar (Tracked) : Tracked_Radar_Block/SC-228 Sensor Model: Radar (Tracked)  dt_s=uas_rdr_trckd_dt_s  lat0_rad=ac1dyn_lat0_rad  lon0_rad=ac1dyn_lon0_rad  alt0_ft=ac1dyn_alt0_ft  sns_for_azimuth_deg=uas_rdr_trckd_sns_for_azimuth_deg  sns_for_elevation_deg=uas_rdr_trckd_sns_for_elevation_deg  debugMode=uas_rdr_trckd_debugMode  rng_random_stddev_ft=uas_rdr_trckd_rng_random_stddev_ft  rng_bias_ft=uas_rdr_trckd_rng_bias_ft  rng_tau_s=uas_rdr_trckd_rng_tau_s  seed1=uas_rdr_trckd_seed1  RCPR_Mode=uas_rdr_trckd_RCPR_Mode  RCPR_Range_ft=uas_rdr_trckd_RCPR_Range_ft  az_random_stddev_rad=uas_rdr_trckd_az_random_stddev_rad  az_bias_rad=uas_rdr_trckd_az_bias_rad  az_tau_s=uas_rdr_trckd_az_tau_s  seed2=uas_rdr_trckd_seed2  el_random_stddev_rad=uas_rdr_trckd_el_random_stddev_rad  el_bias_rad=uas_rdr_trckd_el_bias_rad  el_tau_s=uas_rdr_trckd_el_tau_s  seed3=uas_rdr_trckd_seed3  rngdot_random_stddev_ftps=uas_rdr_trckd_rngdot_random_stddev_ftps  rngdot_bias_ftps=uas_rdr_trckd_rngdot_bias_ftps  rngdot_tau_s=uas_rdr_trckd_rngdot_tau_s  seed4=uas_rdr_trckd_seed4  covRAE=uas_rdr_trckd_reported_errorCovRAE
  Sum : Sum  Inputs=|++
  Sum1 : Sum  Inputs=|++
  Terminator{,1..5} (6 alike) : Terminator
  Transpose : Math  Operator=transpose  SaturateOnIntegerOverflow=on
  sph2cart : sph2cart/sph2cart  SystemSampleTime=-1
      settings: SourceProductName=CASSATTv6: Signals Library
  Intruder AircraftEstimate : Outport
  wires:
  Intruder Aircraft State/1 -> SC-228 Sensor Model: Radar (Tracked)/1
  Intruder Aircraft State Rate/1 -> SC-228 Sensor Model: Radar (Tracked)/2
  SC-228 Sensor Model: Radar (Tracked)/1 -> sph2cart/1  "range"
  sph2cart/8 -> Terminator1/1  "K_FRD"
  SC-228 Sensor Model: Radar (Tracked)/3 -> sph2cart/3  "el_noisy"
  Bus Creator4/1 -> Intruder AircraftEstimate/1  "AircraftEstimate"
  sph2cart/7 -> Terminator/1  "J_FRD"
  SC-228 Sensor Model: Radar (Tracked)/11 -> sph2cart/6  "eldot_rps"
  SC-228 Sensor Model: Radar (Tracked)/9 -> Cast To Boolean/1  "isValid"
  [OwnState] -> Bus Selector/1
  Bus Selector/3 -> NED2FRD/3(phi)  "<phi_rad>"
  Gain3/1 -> Mux3/3
  Constant16/1 -> MATLAB Function/3(h0)
  [OwnState] -> Bus Selector1/1
  sph2cart/2 -> Mux1/2
  Demux/2 -> MATLAB Function/5(e_ft), Bus Creator/2  "e_ft"
  sph2cart/4 -> Mux/1
  SC-228 Sensor Model: Radar (Tracked)/10 -> sph2cart/5  "azdot_rps"
  Bus Selector2/1 -> Mux3/1  "<Ndot_ftps>"
  NaN2/1 -> Bus Creator5/3  "hVar_ft2"
  Demux/1 -> MATLAB Function/4(n_ft), Bus Creator/1  "n_ft"
  sph2cart/1 -> Mux1/1
  Mux3/1 -> Sum1/2
  Demux1/1 -> MATLAB Function/7(vn_ftps), Bus Creator/4  "dn_ftps"
  Mux2/1 -> Sum/2
  Bus Creator/1 -> Bus Creator4/4  "enuStateEstimate"
  Constant15/1 -> MATLAB Function/2(lon0)
  Demux/3 -> Gain/1
  NED2FRD/1(T) -> Transpose/1
  Ownship Aircraft State/1 -> [OwnState], SC-228 Sensor Model: Radar (Tracked)/3
  Demux1/2 -> MATLAB Function/8(ve_ftps), Bus Creator/5  "de_ftps"
  sph2cart/5 -> Mux/2
  NaN5/1 -> Bus Creator5/6  "dhVar_ft2ps2"
  SC-228 Sensor Model: Radar (Tracked)/2 -> sph2cart/2  "az_noisy"
  MATLAB Function/1(lat_rad) -> Bus Creator1/1  "lat_rad"
  SC-228 Sensor Model: Radar (Tracked)/7 -> Terminator4/1
  sph2cart/3 -> Mux1/3
  SC-228 Sensor Model: Radar (Tracked)/5 -> Terminator2/1
  Bus Selector/2 -> NED2FRD/2(theta)  "<theta_rad>"
  Transpose/1 -> Matrix Multiply2/1, Matrix Multiply1/1  "T_F2N"
  Ownship Aircraft State Rate/1 -> [OwnStateRate], SC-228 Sensor Model: Radar (Tracked)/4
  NaN3/1 -> Bus Creator5/4  "dnVar_ft2ps2"
  MATLAB Function/2(lon_rad) -> Bus Creator1/2  "lon_rad"
  Sum/1 -> Demux/1
  NaN/1 -> Bus Creator5/1  "nVar_ft2"
  Bus Selector2/3 -> Gain3/1  "<hdot_ftps>"
  Mux1/1 -> Matrix Multiply1/2
  SC-228 Sensor Model: Radar (Tracked)/6 -> Terminator3/1
  Demux1/3 -> Gain1/1
  Bus Selector1/3 -> Gain2/1  "<h_ft>"
  Bus Selector1/1 -> Mux2/1  "<n_ft>"
  Gain/1 -> MATLAB Function/6(u_ft), Bus Creator/3  "h_ft"
  Gain1/1 -> MATLAB Function/9(vh_ftps), Bus Creator/6  "dh_ftps"
  NaN4/1 -> Bus Creator5/5  "deVar_ft2ps2"
  MATLAB Function/6(dalt_ftps) -> Bus Creator1/6  "dalt_ftps"
  Matrix Multiply2/1 -> Sum1/1
  MATLAB Function/4(dlon_radps) -> Bus Creator1/4  "dlon_radps"
  Mux/1 -> Matrix Multiply2/2
  Clock/1 -> Bus Creator4/2  "timeOfValidity"
  Sum1/1 -> Demux1/1
  Bus Selector2/2 -> Mux3/2  "<Edot_ftps>"
  sph2cart/6 -> Mux/3
  [OwnStateRate] -> Bus Selector2/1
  MATLAB Function/5(alt_ft) -> Bus Creator1/5  "alt_ft"
  Bus Selector/1 -> NED2FRD/1(psi_rad)  "<psi_rad>"
  Bus Selector1/2 -> Mux2/2  "<e_ft>"
  Bus Creator5/1 -> Bus Creator4/5  "covEstimate"
  Bus Creator1/1 -> Bus Creator4/1  "latLonAltEst"
  NaN1/1 -> Bus Creator5/2  "eVar_ft2"
  SC-228 Sensor Model: Radar (Tracked)/4 -> sph2cart/4  "rdot_ftps"
  MATLAB Function/3(dlat_radps) -> Bus Creator1/3  "dlat_radps"
  Matrix Multiply1/1 -> Sum/1
  SC-228 Sensor Model: Radar (Tracked)/8 -> Terminator5/1
  Constant14/1 -> MATLAB Function/1(lat0)
  Gain2/1 -> Mux2/3
  Cast To Boolean/1 -> Bus Creator4/3  "isValid"
